simulink model "test_state"  (R2021a)
settings: Solver=VariableStepAuto  StartTime=0.0  StopTime=inf  RelTol=1e-3
settings Model: EnablePacing=on  Creator=User  LastModifiedBy=User

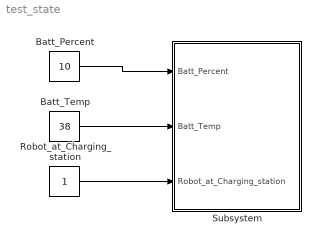
== system test_state ==
  " Batt_Percent" : Constant  Value=10
  " Batt_Temp" : Constant  Value=38
  Robot_at_Charging_station : Constant
  Subsystem : Subsystem
  wires:
  " Batt_Percent"/1 -> Subsystem/1(" Batt_Percent")
  " Batt_Temp"/1 -> Subsystem/2(" Batt_Temp")
  Robot_at_Charging_station/1 -> Subsystem/3(Robot_at_Charging_station)

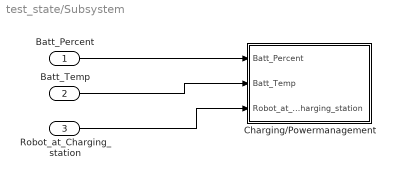
== system test_state/Subsystem ==
  " Batt_Percent" : Inport
  " Batt_Temp" : Inport  Port=2
  Robot_at_Charging_station : Inport  Port=3
  Charging/Powermanagement : Stateflow chart  TreatAsAtomicUnit=on
  wires:
  " Batt_Percent"/1 -> Charging/Powermanagement/1(Batt_Percent)
  " Batt_Temp"/1 -> Charging/Powermanagement/2(Batt_Temp)
  Robot_at_Charging_station/1 -> Charging/Powermanagement/3(Robot_at_Charging_station)

== stateflow chart test_state/Subsystem/Charging//Powermanagement ==
  state standby
    Min_Batt = 20
    move2_C_station = 0
    Batt_Charging_Stat = 0
  state charging
    Max_Batt_Temp = 40
    state check_position_robot_station
      settings: description=Check the position of the robot at the charging station.
    state Start_Batt_Charging
      if Batt_Temp > Max_Batt_Temp
      Batt_Charge_Over_Temp = 1
      end
      settings: description=Check the position of the robot at the charging station.
    state Stop_Batt_Charging
      Batt_Low_Stat = 0
      settings: description=Check the position of the robot at the charging station.
    (default) -> check_position_robot_station : {Batt_Charge_Over_Temp = 0;Emer_Charging = 0}
    check_position_robot_station -> Start_Batt_Charging : [((Robot_at_Charging_station==1&&Batt_Charge_Over_Temp==0)&&Batt_Low_Stat == 1)]{
        | Batt_Charging_Stat = 1}
    Start_Batt_Charging -> Stop_Batt_Charging : [Batt_Percent ==100]{Batt_Charging_Stat = 0}
  state move2goal
  state EmergencyStop
  (default) -> standby
  standby -> charging : [Batt_Percent <= Min_Batt]{Batt_Low_Stat = 1}
  EmergencyStop -> standby : [Batt_Temp < Max_Batt_Temp]
  charging -> standby [order 3] : [Batt_Charging_Stat == 0&&Batt_Low_Stat == 0]{Batt_Low_Stat = 0}
  move2goal -> charging : [Robot_at_Charging_station == 1]
  charging -> move2goal [order 1] : [Robot_at_Charging_station ~= 1]{move2_C_station = 1}
  charging -> EmergencyStop [order 2] : [Batt_Charge_Over_Temp == 1]{Batt_Charging_Stat = 0;Emer_Charging = 1}
  data: Batt_Percent input; Batt_Temp input; Robot_at_Charging_station input; Max_Batt_Temp local; Min_Batt local; move2_C_station local; Batt_Low_Stat local; changing local; Batt_Charging_Stat local; Batt_Charge_Over_Temp local; Chargjng_Emer local; Emer_Charging local
